simulink model "p10"  (R2020a)
settings: Solver=VariableStepAuto  StartTime=0.0  StopTime=10  RelTol=1e-3
model workspace (MAT data in the model file):
  Ia = Simulink.Parameter
  Ia.Value = [0 0 0 0 1]
  Ia.DataType = 'auto'
  Ia.Dimensions = [1 5]
  Vo = Simulink.Parameter
  Vo.Value = [2 4 6 7 8]
  Vo.DataType = 'auto'
  Vo.Dimensions = [1 5]
libraries: simulink x1
settings Model: OrderedModelArguments=off  Creator=007  LastModifiedBy=007

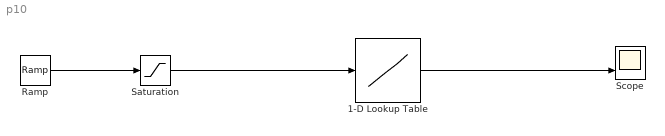
== system p10 ==
  1-D Lookup Table : Lookup_n-D  NumberOfTableDimensions=1  BreakpointsForDimension1=Vo  Table=Ia  InternalRulePriority=Speed  RndMeth=Simplest  InputSameDT=on
  Ramp : simulink/Sources/Ramp  slope=1  start=0  InitialOutput=0
  Saturation : Saturate  UpperLimit=9  LowerLimit=0
  Scope : Scope  NumInputPorts=2
  wires:
  Saturation/1 -> 1-D Lookup Table/1
  Ramp/1 -> Saturation/1
  1-D Lookup Table/1 -> Scope/2
